simulink model "ej_control_pid"  (R2020b)
settings: Solver=VariableStepAuto  StartTime=0.0  StopTime=10  MaxStep=1e-2  RelTol=1e-3
values from neighbouring files (symbols this model uses):
  Kp = 53/4    (= 13.25)    [control_pid.m]    (also in ejemplo_pid.m = 100)
  Td = (51+6)/(4*Kp)    (= 1.07547169811)    [control_pid.m]    (also in ejemplo_pid.m = 0.1)
  Ti = 4*Kp/150    (= 0.353333333333)    [control_pid.m]    (also in ejemplo_pid.m = 0.5)
libraries: pid_lib x1
settings Model: Creator=carma  LastModifiedBy=Acer

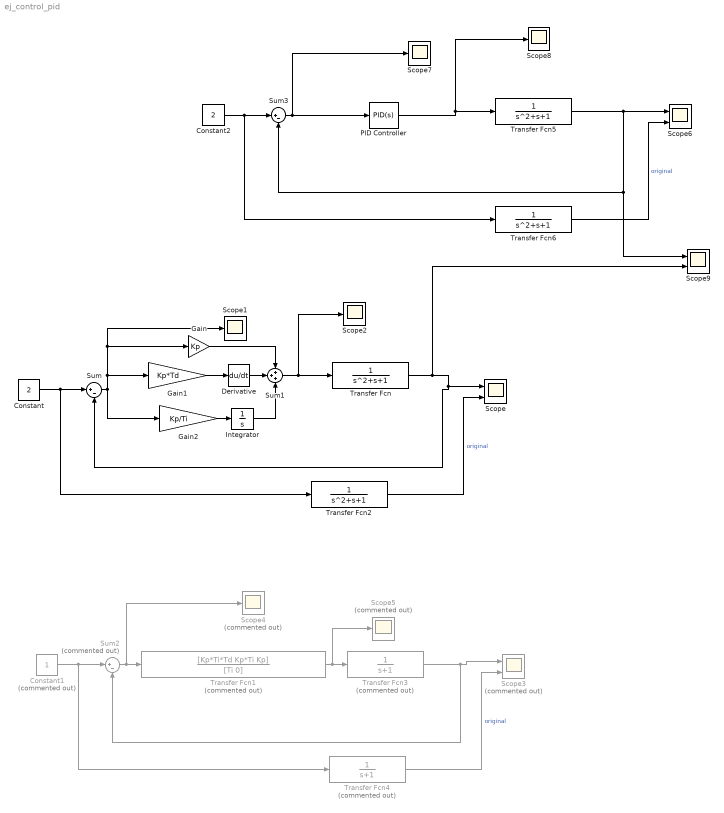
== system ej_control_pid ==
  Constant : Constant  Value=2
  Constant1 : Constant  Commented=on
  Constant2 : Constant  Value=2
  Derivative : Derivative  CoefficientInTFapproximation=0
  Gain : Gain  Gain=Kp
  Gain1 : Gain  Gain=Kp*Td
  Gain2 : Gain  Gain=Kp/Ti
  Integrator : Integrator
  PID Controller : pid_lib/PID Controller  Controller=PID  Form=Parallel  TimeDomain=Continuous-time  UseExternalTs=off  SampleTime=-1  IntegratorMethod=Forward Euler  FilterMethod=Forward Euler  ControllerParametersSource=internal  P=Kp  I=Kp/Ti  D=Kp*Td  UseFilter=on  N=10000  TunerSelectOption=Transfer Function Based (PID Tuner App)  InitialConditionSource=internal  InitialConditionForIntegrator=0  InitialConditionForFilter=0  DifferentiatorICPrevScaledInput=0  ExternalReset=none  TrackingMode=off  Kt=1  LimitOutput=off  SatLimitsSource=internal  UpperSaturationLimit=inf  LowerSaturationLimit=-inf  LinearizeAsGain=on  AntiWindupMode=none  Kb=1  POutMin=[]  POutMax=[]  IOutMin=[]  IOutMax=[]  DOutMin=[]  DOutMax=[]  NOutMin=[]  NOutMax=[]  SumOutMin=[]  SumOutMax=[]  SaturationOutMin=[]  SaturationOutMax=[]  PParamMin=[]  PParamMax=[]  IParamMin=[]  IParamMax=[]  DParamMin=[]  DParamMax=[]  NParamMin=[]  NParamMax=[]  KbParamMin=[]  KbParamMax=[]  KtParamMin=[]  KtParamMax=[]  KbOutMin=[]  KbOutMax=[]  KtOutMin=[]  KtOutMax=[]  IntegratorOutMin=[]  IntegratorOutMax=[]  FilterOutMin=[]  FilterOutMax=[]  SumI1OutMin=[]  SumI1OutMax=[]  SumI2OutMin=[]  SumI2OutMax=[]  SumI3OutMin=[]  SumI3OutMax=[]  SumI4OutMin=[]  SumI4OutMax=[]  SumDOutMin=[]  SumDOutMax=[]  DifferentiatorOutMin=[]  DifferentiatorOutMax=[]  FilterDiffOutCoefMin=[]  FilterDiffOutCoefMax=[]  ReciprocalOutMin=[]  ReciprocalOutMax=[]  SumDenOutMin=[]  SumDenOutMax=[]  SumNumOutMin=[]  SumNumOutMax=[]  DivideOutMin=[]  DivideOutMax=[]  UdiffTsProdOutMin=[]  UdiffTsProdOutMax=[]  NTsProdOutMin=[]  NTsProdOutMax=[]  UintegralTsProdOutMin=[]  UintegralTsProdOutMax=[]  UngainTsProdOutMin=[]  UngainTsProdOutMax=[]  IntegratorContinuousStateAttributes=''  IntegratorStateMustResolveToSignalObject=off  IntegratorRTWStateStorageClass=Auto  FilterContinuousStateAttributes=''  FilterStateMustResolveToSignalObject=off  FilterRTWStateStorageClass=Auto  ParallelPVariant=InternalParameters  IdealPVariant=Disabled  IVariant=InternalParameters  DVariant=InternalParameters  IntegratorVariant=Continuous  SatVariant=Disabled  AWVariant=Passthrough  PCopyVariant=Disabled  TRVariant=Disabled  FdbkBlocksVariant=Forward  IdealPFdbkVariant=Disabled  SatFdbkVariant=Disabled  DerivativeFilterVariant=ContFilter  NVariant=InternalParameters  NCopyVariant=Disabled  FilterICVariant=InternalICsFilter  IntegratorICVariant=InternalICs  ExternalResetVariant=Disabled  TRSumVariant=Passthrough  SumFdbkVariant=Disabled  SumVariant=Sum_PID  TsampFilterVariant=InternalTs  TsampNgainVariant=Passthrough  TsampIntegralVariant=Passthrough  ExternalSaturationOutDataTypeStr=Inherit: Same as second input
  Scope : Scope  NumInputPorts=2
  Scope{1..2,7..8} (4 alike) : Scope
  Scope3 : Scope  Commented=on  NumInputPorts=2
  Scope4 : Scope  Commented=on
  Scope5 : Scope  Commented=on
  Scope6 : Scope  NumInputPorts=2
  Scope9 : Scope  NumInputPorts=2
  Sum : Sum  Inputs=|+-
  Sum1 : Sum  Inputs=+++
  Sum2 : Sum  Commented=on  Inputs=|+-
  Sum3 : Sum  Inputs=|+-
  Transfer Fcn{,2,5..6} (4 alike) : TransferFcn  Denominator=[1 1 1]
  Transfer Fcn1 : TransferFcn  Commented=on  Numerator=[Kp*Ti*Td Kp*Ti Kp]  Denominator=[Ti 0]
  Transfer Fcn3 : TransferFcn  Commented=on  Denominator=[1 1]
  Transfer Fcn4 : TransferFcn  Commented=on  Denominator=[1 1]
  wires:
  Constant/1 -> Transfer Fcn2/1, Sum/1
  Sum/1 -> Gain1/1, Gain/1, Scope1/1, Gain2/1
  Sum1/1 -> Scope2/1, Transfer Fcn/1
  Transfer Fcn/1 -> Scope9/2, Sum/2, Scope/1
  Gain/1 -> Sum1/1
  Transfer Fcn2/1 -> Scope/2  "original"
  Gain2/1 -> Integrator/1
  Integrator/1 -> Sum1/3
  Gain1/1 -> Derivative/1
  Derivative/1 -> Sum1/2
  Sum2/1 -> Transfer Fcn1/1, Scope4/1
  Constant1/1 -> Transfer Fcn4/1, Sum2/1
  Transfer Fcn4/1 -> Scope3/2  "original"
  Transfer Fcn3/1 -> Scope3/1, Sum2/2
  Transfer Fcn1/1 -> Scope5/1, Transfer Fcn3/1
  PID Controller/1 -> Scope8/1, Transfer Fcn5/1
  Transfer Fcn5/1 -> Scope9/1, Sum3/2, Scope6/1
  Transfer Fcn6/1 -> Scope6/2  "original"
  Sum3/1 -> PID Controller/1, Scope7/1
  Constant2/1 -> Transfer Fcn6/1, Sum3/1
